simulink model "ramp_constant"  (R2021b)
settings: Solver=VariableStepAuto  StartTime=0.0  StopTime=10  RelTol=1e-3
libraries: simulink x2
settings Model: Creator=28626  LastModifiedBy=28626

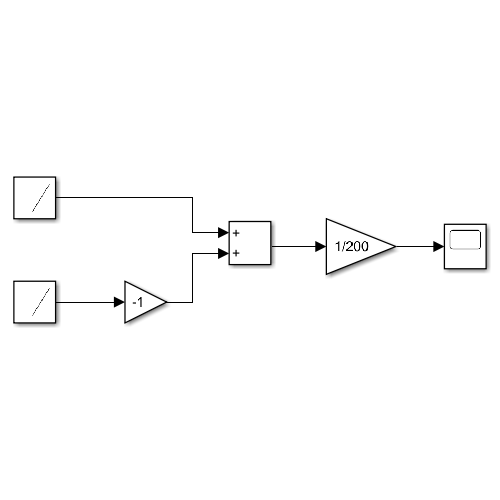
[thumbnail: Simulink's stored preview of the top-level diagram]
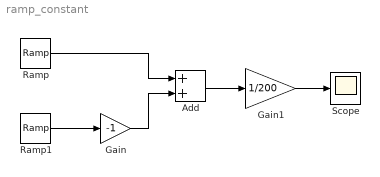
== system ramp_constant ==
  Add : Sum
  Gain : Gain  Gain=-1
  Gain1 : Gain  Gain=1/200
  Ramp : simulink/Sources/Ramp  slope=600000000  start=0  InitialOutput=0
  Ramp1 : simulink/Sources/Ramp  slope=600000000  start=7  InitialOutput=0
  Scope : Scope
  wires:
  Ramp/1 -> Add/1
  Ramp1/1 -> Gain/1
  Gain/1 -> Add/2
  Add/1 -> Gain1/1
  Gain1/1 -> Scope/1
